simulink model "task_1_2"  (R2023a)
settings: Solver=VariableStepAuto  StartTime=0.0  StopTime=10.0  RelTol=1e-8
settings Model: Creator=user  LastModifiedBy=user

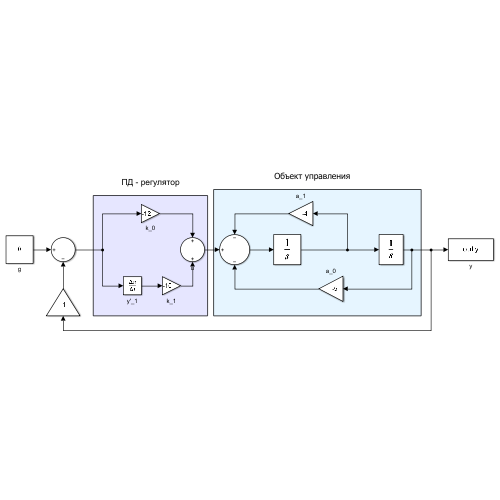
[thumbnail: Simulink's stored preview of the top-level diagram]
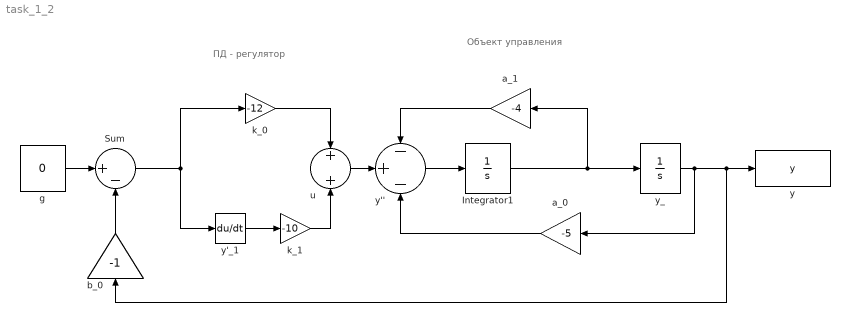
== system task_1_2 ==
  note: Объект управления
  note: ПД - регулятор
  Integrator1 : Integrator  InitialCondition=1
  Sum : Sum  Inputs=|+-
  a_0 : Gain  Gain=-5
  a_1 : Gain  Gain=-4
  b_0 : Gain  Gain=-1
  g : Constant  Value=0
  k_0 : Gain  Gain=-12
  k_1 : Gain  Gain=-10
  u : Sum
  y : ToWorkspace  VariableName=y  SaveFormat=Timeseries  SampleTime=-1
  y'' : Sum  Inputs=-+-
  y'_1 : Derivative
  y_ : Integrator  InitialCondition=1
  wires:
  a_0/1 -> y''/3
  y''/1 -> Integrator1/1
  Integrator1/1 -> a_1/1, y_/1
  u/1 -> y''/2
  k_0/1 -> u/1
  k_1/1 -> u/2
  y'_1/1 -> k_1/1
  a_1/1 -> y''/1
  g/1 -> Sum/1
  b_0/1 -> Sum/2
  y_/1 -> b_0/1, y/1, a_0/1
  Sum/1 -> y'_1/1, k_0/1
